simulink model "pipeline_13bit"  (R2021b)
settings: Solver=FixedStepDiscrete  StartTime=0.0  StopTime=5000*ts  FixedStep=ts  RelTol=1e-3
undefined symbols (not defined in the file): fin, ts
(part 2 of 2)

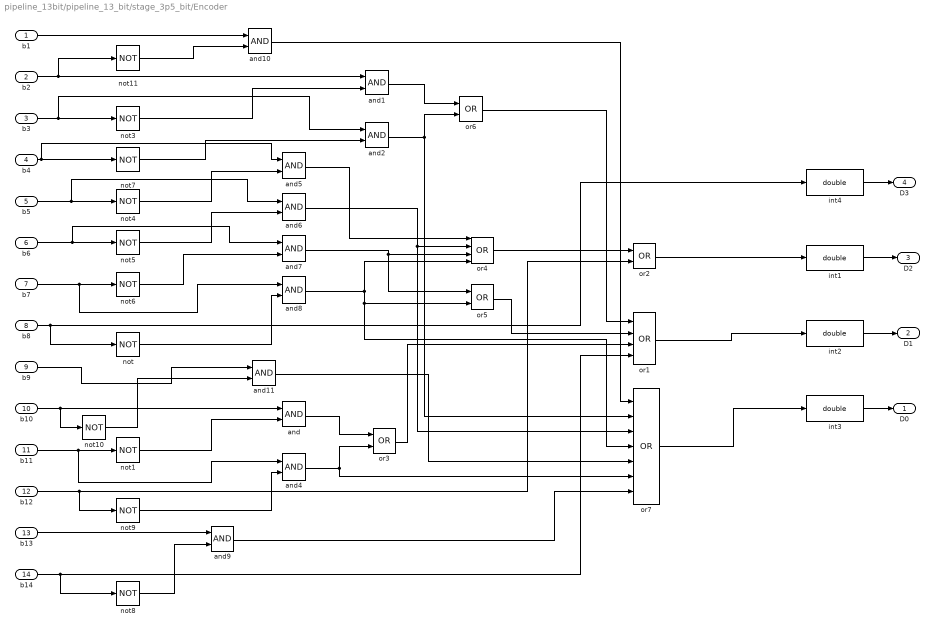
== system pipeline_13bit/pipeline_13_bit/stage_3p5_bit/Encoder ==
  b1 : Inport
  b2 : Inport  Port=2
  b3 : Inport  Port=3
  b4 : Inport  Port=4
  b5 : Inport  Port=5
  b6 : Inport  Port=6
  b7 : Inport  Port=7
  b8 : Inport  Port=8
  b9 : Inport  Port=9
  b10 : Inport  Port=10
  b11 : Inport  Port=11
  b12 : Inport  Port=12
  b13 : Inport  Port=13
  b14 : Inport  Port=14
  and{,1..2,4..11} (11 alike) : Logic  AllPortsSameDT=off  OutDataTypeStr=boolean
  int{1..4} (4 alike) : DataTypeConversion  OutDataTypeStr=double
  not{,1,3..11} (11 alike) : Logic  Operator=NOT  AllPortsSameDT=off  OutDataTypeStr=boolean
  or1 : Logic  Operator=OR  Inputs=4  AllPortsSameDT=off  OutDataTypeStr=boolean
  or{2..3,5..6} (4 alike) : Logic  Operator=OR  AllPortsSameDT=off  OutDataTypeStr=boolean
  or4 : Logic  Operator=OR  Inputs=4  AllPortsSameDT=off  OutDataTypeStr=boolean
  or7 : Logic  Operator=OR  Inputs=7  AllPortsSameDT=off  OutDataTypeStr=boolean
  D0 : Outport
  D1 : Outport  Port=2
  D2 : Outport  Port=3
  D3 : Outport  Port=4
  wires:
  int2/1 -> D1/1
  int3/1 -> D0/1
  int1/1 -> D2/1
  int4/1 -> D3/1
  b8/1 -> int4/1, not/1
  b12/1 -> not9/1, or2/2
  b5/1 -> and6/1, not4/1
  b6/1 -> and7/1, not5/1
  b7/1 -> and8/1, not6/1
  and8/1 -> or7/4, or5/2, or4/4
  and7/1 -> or5/1, or4/3
  and6/1 -> or7/3, or4/2
  and5/1 -> or4/1
  or4/1 -> or2/1
  or2/1 -> int1/1
  b14/1 -> not8/1, or1/4
  b10/1 -> not10/1, and/1
  b11/1 -> and4/1, not1/1
  not1/1 -> and/2
  b4/1 -> not7/1, and5/1
  not4/1 -> and5/2
  not5/1 -> and6/2
  not6/1 -> and7/2
  not/1 -> and8/2
  and/1 -> or3/1
  and4/1 -> or7/6, or3/2
  or3/1 -> or1/3
  or5/1 -> or1/2
  b3/1 -> and2/1, not3/1
  b2/1 -> not11/1, and1/1
  not3/1 -> and1/2
  or1/1 -> int2/1
  not7/1 -> and2/2
  and1/1 -> or6/1
  and2/1 -> or7/2, or6/2
  or6/1 -> or1/1
  or7/1 -> int3/1
  b13/1 -> and9/1
  not8/1 -> and9/2
  and9/1 -> or7/7
  not9/1 -> and4/2
  b9/1 -> and11/1
  not10/1 -> and11/2
  and11/1 -> or7/5
  b1/1 -> and10/1
  not11/1 -> and10/2
  and10/1 -> or7/1

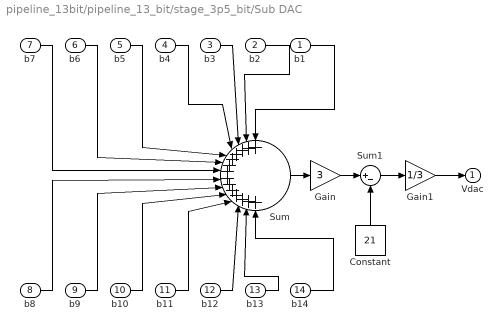
== system pipeline_13bit/pipeline_13_bit/stage_3p5_bit/Sub DAC ==
  b1 : Inport
  b2 : Inport  Port=2
  b3 : Inport  Port=3
  b4 : Inport  Port=4
  b5 : Inport  Port=5
  b6 : Inport  Port=6
  b7 : Inport  Port=7
  b8 : Inport  Port=8
  b9 : Inport  Port=9
  b10 : Inport  Port=10
  b11 : Inport  Port=11
  b12 : Inport  Port=12
  b13 : Inport  Port=13
  b14 : Inport  Port=14
  Constant : Constant  Value=21
  Gain : Gain  Gain=3
  Gain1 : Gain  Gain=1/3
  Sum : Sum  Inputs=++++++++++++++
  Sum1 : Sum  Inputs=|+-
  Vdac : Outport
  wires:
  b1/1 -> Sum/1
  b2/1 -> Sum/2
  b3/1 -> Sum/3
  b4/1 -> Sum/4
  b5/1 -> Sum/5
  b6/1 -> Sum/6
  Sum/1 -> Gain/1
  Gain/1 -> Sum1/1
  Constant/1 -> Sum1/2
  Sum1/1 -> Gain1/1
  Gain1/1 -> Vdac/1
  b7/1 -> Sum/7
  b8/1 -> Sum/8
  b9/1 -> Sum/9
  b10/1 -> Sum/10
  b11/1 -> Sum/11
  b12/1 -> Sum/12
  b13/1 -> Sum/13
  b14/1 -> Sum/14
